simulink model "DCMotorMPC"  (R2022b)
settings: Solver=ode45  StartTime=0.0  StopTime=2.5  FixedStep=1e-4  RelTol=1e-3
libraries: eePwmGenerator x1
settings Model: Creator=Ananda Tjakra  LastModifiedBy=anand
settings SolverCC: AlgebraicLoopSolver=TrustRegion
settings DebuggingCC: UnconnectedInputMsg=warning  UnconnectedOutputMsg=warning  UnconnectedLineMsg=warning  SFMachineParentedDataDiag=warning
settings ModelReferenceCC: EnableRefExpFcnMdlSchedulingChecks=on

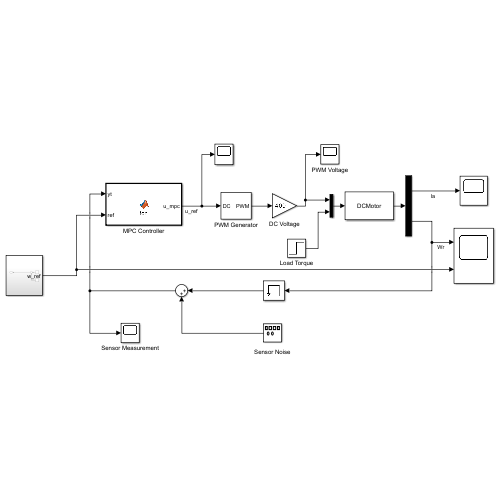
[thumbnail: Simulink's stored preview of the top-level diagram]
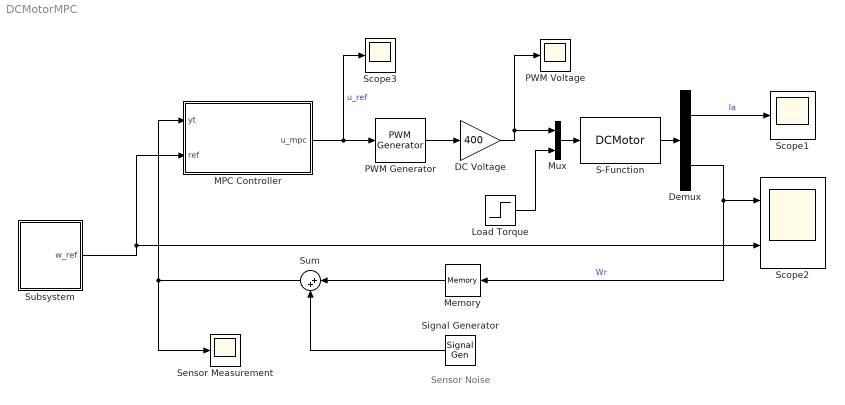
== system DCMotorMPC ==
  note: Sensor Noise
  DC Voltage : Gain  Gain=400
  Demux : Demux  Outputs=2
  Load Torque : Step  After=3  SampleTime=0
  MPC Controller : MATLAB Function  TreatAsAtomicUnit=on
  Memory : Memory
  Mux : Mux  Inputs=2
  PWM Generator : eePwmGenerator/PWM Generator  CarrCount=Up  Tper=0.001  Tdelay=0  Ts=1e-4
  PWM Voltage : Scope
  S-Function : S-Function  FunctionName=DCMotor  SFunctionDeploymentMode=off  EnableBusSupport=off
  Scope1 : Scope
  Scope2 : Scope  NumInputPorts=2
  Scope3 : Scope
  Sensor Measurement : Scope
  Signal Generator : SignalGenerator  WaveForm=random  Amplitude=0
  Subsystem : Subsystem
  Sum : Sum  Inputs=|++
  wires:
  Demux/2 -> Memory/1, Scope2/1  "Wr"
  Demux/1 -> Scope1/1  "Ia"
  S-Function/1 -> Demux/1
  Subsystem/1(w_ref) -> MPC Controller/2(ref), Scope2/2
  Memory/1 -> Sum/1
  Sum/1 -> Sensor Measurement/1, MPC Controller/1(yt)
  Signal Generator/1 -> Sum/2
  MPC Controller/1(u_mpc) -> PWM Generator/1, Scope3/1  "u_ref"
  PWM Generator/1 -> DC Voltage/1
  DC Voltage/1 -> Mux/1, PWM Voltage/1
  Mux/1 -> S-Function/1
  Load Torque/1 -> Mux/2

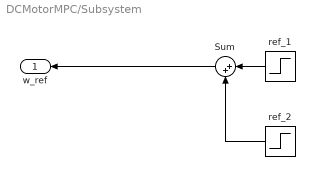
== system DCMotorMPC/Subsystem ==
  Sum : Sum  Inputs=|++
  ref_1 : Step  Time=0.5  After=400  SampleTime=0
  ref_2 : Step  Time=1.5  After=200  SampleTime=0
  w_ref : Outport
  wires:
  ref_1/1 -> Sum/1
  ref_2/1 -> Sum/2
  Sum/1 -> w_ref/1

== matlab function DCMotorMPC/MPC Controller ==
  data: u_mpc output; yt input; ref input
function u_mpc = fcn(yt,ref)

% System discrete model at Ts = 1e-4
Ad = [0.999078612745286	-0.000105301249844195;...
2.45332729742468e-05	0.999999942082396];
Bd = [8.22666037703133e-05;1.00975483059156e-09];
Cd = [0 1];
Dd = [0];

% Input and Output Calculation
n=size(Ad,1);
p=size(Bd,2);

% Controller and Gradient Descent Parameter
R = 0.00002*eye(10);
Q = 50*eye(10);
Np = 10; % Prediction Horizon
alpha=10; % Step Size

% Reference Signal
rp = ref*ones(Np,1);

% Matrix Augmentation for Observer
Aa=[Ad zeros(n,p);Cd*Ad eye(p)];
Ba=[Bd;Cd*Bd];
Ca=[zeros(n,p)' eye(p)];


% Observer Matrix for Np = 10
W=[Ca*Aa;Ca*(Aa^2);Ca*(Aa^3);Ca*(Aa^4);Ca*(Aa^5);Ca*(Aa^6);Ca*(Aa^7);...
    Ca*(Aa^8);Ca*(Aa^9);Ca*(Aa^10);];

Z=[Ca*Ba 0 0 0 0 0 0 0 0 0;...
    Ca*Aa*Ba Ca*Ba 0 0 0 0 0 0 0 0;...
    Ca*(Aa^2)*Ba Ca*Aa*Ba Ca*Ba 0 0 0 0 0 0 0;...
    Ca*(Aa^3)*Ba Ca*(Aa^2)*Ba Ca*Aa*Ba Ca*Ba 0 0 0 0 0 0;...
    Ca*(Aa^4)*Ba Ca*(Aa^3)*Ba Ca*(Aa^2)*Ba Ca*Aa*Ba Ca*Ba 0 0 0 0 0;...
    Ca*(Aa^5)*Ba Ca*(Aa^4)*Ba Ca*(Aa^3)*Ba Ca*(Aa^2)*Ba Ca*Aa*Ba Ca*Ba 0 0 0 0;...
    Ca*(Aa^6)*Ba Ca*(Aa^5)*Ba Ca*(Aa^4)*Ba Ca*(Aa^3)*Ba Ca*(Aa^2)*Ba Ca*Aa*Ba Ca*Ba 0 0 0;...
    Ca*(Aa^7)*Ba Ca*(Aa^6)*Ba Ca*(Aa^5)*Ba Ca*(Aa^4)*Ba Ca*(Aa^3)*Ba Ca*(Aa^2)*Ba Ca*Aa*Ba Ca*Ba 0 0;...
    Ca*(Aa^8)*Ba Ca*(Aa^7)*Ba Ca*(Aa^6)*Ba Ca*(Aa^5)*Ba Ca*(Aa^4)*Ba Ca*(Aa^3)*Ba Ca*(Aa^2)*Ba Ca*Aa*Ba Ca*Ba 0;...
    Ca*(Aa^9)*Ba Ca*(Aa^8)*Ba Ca*(Aa^7)*Ba Ca*(Aa^6)*Ba Ca*(Aa^5)*Ba Ca*(Aa^4)*Ba Ca*(Aa^3)*Ba Ca*(Aa^2)*Ba Ca*Aa*Ba Ca*Ba];

% Initial States and input [del_x_1;del_x_2;z_k] and del_u
xa=zeros(n+p,p);
xa(3) = yt;
Del_U=zeros(Np,1);

% Gradient Descent Method
Max_Iter=1e4;  
    %Gradient Descent
    for i=1:Max_Iter    
         grad_J=-(rp-W*xa-Z*Del_U)'*Q*Z + Del_U'*R;
         Del_U = Del_U - (alpha)*(grad_J');
    end

%Output Computation with u_ref=del_u(1)
u_mpc = Del_U(1);
u_mpc = u_mpc/400;
